simulink library "model_library"  (R2016b)
settings: Solver=ode45  StartTime=0.0  StopTime=10.0  RelTol=1e-3  EnableMultiTasking=on
libraries: model_library x2
settings Model: Creator=zjiang  LastModifiedBy=jangkj
settings DataIOCC: LimitDataPoints=on  SaveFormat=Array
settings OptimizationCC: LifeSpan=inf
settings DebuggingCC: SolverPrmCheckMsg=warning  SFUnexpectedBacktrackingDiag=warning  SFNoUnconditionalDefaultTransitionDiag=warning  SFExecutionAtInitializationDiag=none
settings HardwareCC: ProdBitPerPointer=32  ProdBitPerSizeT=32  ProdBitPerPtrDiffT=32  ProdLargestAtomicFloat=None  ProdIntDivRoundTo=Undefined  ProdEndianess=Unspecified  ProdWordSize=32  ProdHWDeviceType=32-bit Generic
settings ModelReferenceCC: PropagateSignalLabelsOutOfModel=off
settings GRTTargetCC: TargetLangStandard=C89/C90 (ANSI)  GeneratePreprocessorConditionals=Disable all
settings ConfigComp: CovMetricSettings=dw  CovHtmlReporting=on  CovSaveCumulativeToWorkspaceVar=on  CovSaveSingleToWorkspaceVar=on  CovExternalEMLEnable=off  CovSFcnEnable=off

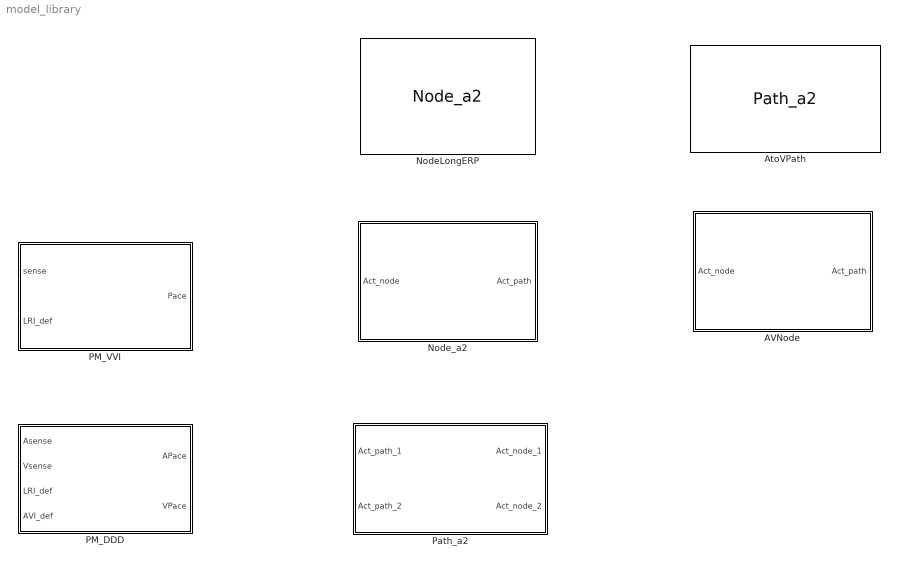
== system model_library ==
  AVNode : Subsystem  AncestorBlock=model_library/Node_a2
  AtoVPath : model_library/Path_a2
      link override Tcond_def: Value=150
  NodeLongERP : model_library/Node_a2
      link override ERP_def: Value=11
      link override Rest_def: Value=22
  Node_a2 : Subsystem  AncestorBlock=model_library/Node_a1
  PM_DDD : Stateflow chart  TreatAsAtomicUnit=on
  PM_VVI : Stateflow chart  TreatAsAtomicUnit=on
  Path_a2 : Subsystem  AncestorBlock=model_library/Path_a3

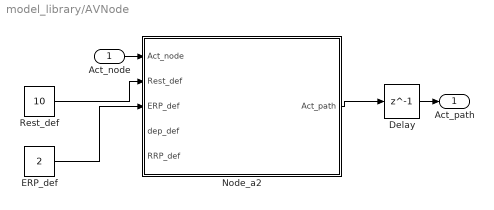
== system model_library/AVNode ==
  Act_node : Inport
  Delay : Delay  DelayLength=1  InitialCondition=0
  ERP_def : Constant  Value=2  OutDataTypeStr=uint16
  Node_a2 : Stateflow chart  RequirementInfo="{}  %GIDa_6ee29377_7781_44c0_ad76_b00d26592997"  TreatAsAtomicUnit=on
  Rest_def : Constant  Value=10  OutDataTypeStr=uint16
  Act_path : Outport
  wires:
  Node_a2/1(Act_path) -> Delay/1
  Act_node/1 -> Node_a2/1(Act_node)
  Rest_def/1 -> Node_a2/2(Rest_def)
  ERP_def/1 -> Node_a2/3(ERP_def)
  Delay/1 -> Act_path/1

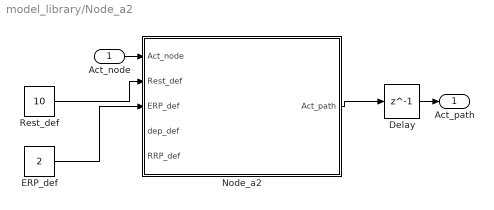
== system model_library/Node_a2 ==
  Act_node : Inport
  Delay : Delay  DelayLength=1  InitialCondition=0
  ERP_def : Constant  Value=2  OutDataTypeStr=uint16
  Node_a2 : Stateflow chart  RequirementInfo="{}  %GIDa_6ee29377_7781_44c0_ad76_b00d26592997"  TreatAsAtomicUnit=on
  Rest_def : Constant  Value=10  OutDataTypeStr=uint16
  Act_path : Outport
  wires:
  Node_a2/1(Act_path) -> Delay/1
  Act_node/1 -> Node_a2/1(Act_node)
  Rest_def/1 -> Node_a2/2(Rest_def)
  ERP_def/1 -> Node_a2/3(ERP_def)
  Delay/1 -> Act_path/1

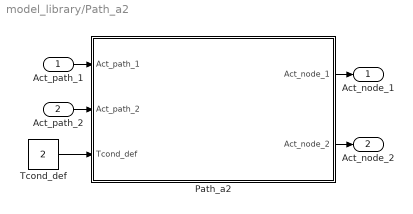
== system model_library/Path_a2 ==
  Act_path_1 : Inport
  Act_path_2 : Inport  Port=2
  Path_a2 : Stateflow chart  TreatAsAtomicUnit=on
  Tcond_def : Constant  Value=2  OutDataTypeStr=uint16
  Act_node_1 : Outport
  Act_node_2 : Outport  Port=2
  wires:
  Path_a2/1(Act_node_1) -> Act_node_1/1
  Act_path_2/1 -> Path_a2/2(Act_path_2)
  Act_path_1/1 -> Path_a2/1(Act_path_1)
  Path_a2/2(Act_node_2) -> Act_node_2/1
  Tcond_def/1 -> Path_a2/3(Tcond_def)

== stateflow chart model_library/PM_VVI ==
  state Pm
    state LRI
    state temp
      du:uptime_p = uptime_p + 1;
      du:LRI_cur = LRI_cur - 1;
    (default) -> LRI : {LRI_cur=LRI_def;Pace=false;}
    LRI -> LRI [order 1] : [sense==false && LRI_cur>0]/{LRI_cur = LRI_cur - 1;}
    LRI -> LRI [order 3] : [sense==true]/{LRI_cur=LRI_def;}
    temp -> LRI : [uptime_p>=3]/{Pace=false;}
    LRI -> temp [order 2] : [sense==0 && LRI_cur<=0]/{LRI_cur=LRI_def;Pace=true;uptime_p= uint16(0);}
  data: sense input boolean; Pace output boolean; uptime_p local uint16; LRI_def input uint16; LRI_cur local uint16

== stateflow chart model_library/PM_DDD ==
  state PM
    state LRI
    state ap
      du:uptime_p = uptime_p + 1;
      du:AVI_cur = AVI_cur - 1;
    state AVI
      du:AVI_cur=AVI_cur-1;
    state vp
      du:uptime_p = uptime_p + 1;
      du:LRI_cur = LRI_cur - 1;
    (default) -> LRI : {LRI_cur=LRI_def;AVI_cur=AVI_def;APace=false;VPace=false;}
    LRI -> ap [order 2] : [Asense==false && Vsense==false && LRI_cur<AVI_def]/{APace=true;AVI_cur=AVI_def;uptime_p=uint16(0);}
    LRI -> LRI [order 1] : [Vsense==true]/{LRI_cur=LRI_def;}
    LRI -> AVI [order 3] : [Asense==true]/{AVI_cur=AVI_def;}
    LRI -> LRI [order 4] : [Asense==false && Vsense==false && LRI_cur>=AVI_def]/{LRI_cur = LRI_cur - 1;}
    ap -> AVI : [uptime_p>0]/{APace=false;}
    vp -> LRI : [uptime_p>0]/{VPace=false;}
    AVI -> LRI [order 2] : [Vsense==true]/{LRI_cur=LRI_def;}
    AVI -> vp [order 1] : [Asense==false && Vsense==false && AVI_cur<=0]/{LRI_cur=LRI_def;VPace=true;uptime_p= uint16(0);}
  data: Asense input boolean; Vsense input boolean; APace output boolean; uptime_p local uint16; LRI_def input uint16; LRI_cur local uint16; VPace output boolean; AVI_cur local uint16; AVI_def input uint16

== stateflow chart model_library/Node_a2/Node_a2 ==
  state node
    settings: description=|
        | temp can be thought of a sub-mode of ERP, which only exists to make sure that act_path is high for one period.
        | 
        | In ERP, if Act_node is received, then it is ignored through that self-transition.
        | 
        | Note this doesn't model variations in cycle length because everytime it is stimulated in RRP, ERP_cur is set to ERP_def again.
    state Rest
    state RRP
    state ERP
    state temp
    (default) -> Rest : {Rest_cur=Rest_def;}
    Rest -> temp [order 3] : [Act_node==false && Rest_cur<=uint16(0)]/{Act_path=true;uptime= uint16(0);ERP_cur=ERP_def;}
    Rest -> temp [order 1] : [Act_node==true]/{Act_path=true;uptime= uint16(0);ERP_cur=ERP_def;}
    Rest -> Rest [order 2] : [Act_node==false && Rest_cur>uint16(0)]/{Rest_cur = Rest_cur - uint16(1);}
    RRP -> Rest [order 1] : [RRP_cur<=0]/{Rest_cur=Rest_def;}
    RRP -> RRP [order 2] : [Act_node==false && RRP_cur>0]/{RRP_cur=RRP_cur-uint16(1);}
    RRP -> temp [order 3] : [Act_node==true]/{Act_path=true;uptime= uint16(0);ERP_cur=ERP_def;}
    ERP -> RRP [order 1] : [ERP_cur<=uint16(0)]/{RRP_cur=RRP_def;}
    temp -> temp [order 1] : [uptime<uint16(1)]/{uptime = uptime + uint16(1);ERP_cur =ERP_cur - uint16(1);}
    temp -> ERP [order 2] : [uptime>=uint16(1)]/{Act_path=false;}
    ERP -> ERP [order 3] : [Act_node==true]
    ERP -> ERP [order 2] : {ERP_cur = ERP_cur - uint16(1);}
  data: Act_node input boolean; Act_path output boolean; Rest_cur local uint16; ERP_cur local uint16; Rest_def input uint16; ERP_def input uint16; uptime local uint16; dep_cur local uint16; dep_def input uint16; RRP_cur local uint16; RRP_def input uint16

== stateflow chart model_library/Path_a2/Path_a2 ==
  state path
    state Idle
    state Ante
    state Retro
    state Wait
    state Double
    (default) -> Idle
    Idle -> Ante [order 1] : [Act_path_1==true]/{Tcond_cur=Tcond_def;}
    Idle -> Retro [order 2] : [Act_path_2==true]/{Tcond_cur=Tcond_def;}
    Wait -> Idle [order 1] : [uptime>0]/{Act_node_1=false;Act_node_2=false;}
    Ante -> Ante [order 3] : [Act_path_2==false && Tcond_cur>uint16(0)]/{Tcond_cur = Tcond_cur - uint16(1);}
    Retro -> Retro [order 3] : [Act_path_1==false && Tcond_cur>uint16(0)]/{Tcond_cur = Tcond_cur - uint16(1);}
    Ante -> Double [order 2] : [Act_path_2==true]
    Ante -> Wait [order 1] : [Act_path_2==false && Tcond_cur<=uint16(0)]/{Act_node_2=true;uptime=uint16(0);}
    Retro -> Double [order 2] : [Act_path_1==true]
    Retro -> Wait [order 1] : [Act_path_1==false && Tcond_cur<=uint16(0)]/{Act_node_1=true;uptime=uint16(0);}
    Wait -> Wait [order 2] : [uptime<=uint16(0)]/{uptime = uptime + uint16(1);}
    Double -> Wait [order 1] : [Tcond_cur<=uint16(0)]/{uptime=uint16(0);}
    Double -> Double [order 2] : [Tcond_cur>uint16(0)]/{Tcond_cur=Tcond_cur-uint16(1);}
  data: Act_path_1 input boolean; Act_path_2 input boolean; Act_node_1 output boolean; Act_node_2 output boolean; Tcond_cur local uint16; Tcond_def input uint16; uptime local uint16

== stateflow chart model_library/AVNode/Node_a2 ==
  state node
    settings: description=|
        | temp can be thought of a sub-mode of ERP, which only exists to make sure that act_path is high for one period.
        | 
        | In ERP, if Act_node is received, then it is ignored through that self-transition.
        | 
        | Note this doesn't model variations in cycle length because everytime it is stimulated in RRP, ERP_cur is set to ERP_def again.
    state Rest
    state RRP
    state ERP
    state temp
    (default) -> Rest : {Rest_cur=Rest_def;}
    Rest -> temp [order 3] : [Act_node==false && Rest_cur<=uint16(0)]/{Act_path=true;uptime= uint16(0);ERP_cur=ERP_def;}
    Rest -> temp [order 1] : [Act_node==true]/{Act_path=true;uptime= uint16(0);ERP_cur=ERP_def;}
    Rest -> Rest [order 2] : [Act_node==false && Rest_cur>uint16(0)]/{Rest_cur = Rest_cur - uint16(1);}
    RRP -> Rest [order 1] : [RRP_cur<=0]/{Rest_cur=Rest_def;}
    RRP -> RRP [order 2] : [Act_node==false && RRP_cur>0]/{RRP_cur=RRP_cur-uint16(1);}
    RRP -> temp [order 3] : [Act_node==true]/{Act_path=true;uptime= uint16(0);ERP_cur=ERP_def;}
    ERP -> RRP [order 1] : [ERP_cur<=uint16(0)]/{RRP_cur=RRP_def;}
    temp -> temp [order 1] : [uptime<uint16(1)]/{uptime = uptime + uint16(1);ERP_cur =ERP_cur - uint16(1);}
    temp -> ERP [order 2] : [uptime>=uint16(1)]/{Act_path=false;}
    ERP -> ERP [order 3] : [Act_node==true]
    ERP -> ERP [order 2] : {ERP_cur = ERP_cur - uint16(1);}
  data: Act_node input boolean; Act_path output boolean; Rest_cur local uint16; ERP_cur local uint16; Rest_def input uint16; ERP_def input uint16; uptime local uint16; dep_cur local uint16; dep_def input uint16; RRP_cur local uint16; RRP_def input uint16
